simulink model "Coupled_Model_crosslinked_intext"  (R2016a)
settings: Solver=FixedStepDiscrete  StartTime=0  StopTime=1000  FixedStep=1  RelTol=1e-3
undefined symbols (not defined in the file or in its folder): DiscIntNeverNeededParam
libraries: simulink_extras x32
(part 2 of 3)

== system Coupled_Model_crosslinked_intext/kMtcontrol/kMtcontrol3/kMt Dynamics ==
  Fk : Inport
  Add : Sum  Inputs=-+
  Add1 : Sum  Inputs=-+
  Add2 : Sum
  Discrete-Time Integrator : DiscreteIntegrator  InitialConditionSource=external  ICPrevOutput=DiscIntNeverNeededParam  ICPrevScaledInput=DiscIntNeverNeededParam
  Discrete-Time Integrator1 : DiscreteIntegrator  InitialConditionSource=external  ICPrevOutput=DiscIntNeverNeededParam  ICPrevScaledInput=DiscIntNeverNeededParam
  Mux : Mux  Inputs=2
  Product{1..4} (4 alike) : Product  RndMeth=Zero
  kMtState : Subsystem
  LkMt : Outport
  tag scope: kMt13=global
  wires:
  Fk/1 -> kMtState/2(Fspr)
  kMtState/2(RLeft) -> Product2/1
  Product1/1 -> Add/1
  Product2/1 -> Add/2
  Product3/1 -> Add1/2
  Product4/1 -> Add1/1
  kMtState/4(RRight) -> Product3/1
  kMtState/1(CLeft) -> Product1/1
  Add/1 -> Discrete-Time Integrator/1  "glkMt"
  Add1/1 -> Discrete-Time Integrator1/1  "grkMt"
  Discrete-Time Integrator1/1 -> Add2/2, kMtState/3(LrkMt), Mux/2
  Discrete-Time Integrator/1 -> Add2/1, kMtState/1(LlkMt), Mux/1
  Add2/1 -> LkMt/1
  kMtState/3(CRight) -> Product4/1
  [Rgro] -> Product2/2, Product3/2
  [Rshr] -> Product1/2, Product4/2
  Mux/1 -> [kMt13]
  [LkMt] -> Discrete-Time Integrator/2
  [LkMt] -> Discrete-Time Integrator1/2

== system Coupled_Model_crosslinked_intext/kMtcontrol/kMtcontrol3/kMt Dynamics  ==
  Fk : Inport
  Add : Sum  Inputs=-+
  Add1 : Sum  Inputs=-+
  Add2 : Sum
  Discrete-Time Integrator : DiscreteIntegrator  InitialConditionSource=external  ICPrevOutput=DiscIntNeverNeededParam  ICPrevScaledInput=DiscIntNeverNeededParam
  Discrete-Time Integrator1 : DiscreteIntegrator  InitialConditionSource=external  ICPrevOutput=DiscIntNeverNeededParam  ICPrevScaledInput=DiscIntNeverNeededParam
  Mux : Mux  Inputs=2
  Product{1..4} (4 alike) : Product  RndMeth=Zero
  kMtState : Subsystem
  LkMt : Outport
  tag scope: kMt14=global
  wires:
  Fk/1 -> kMtState/2(Fspr)
  kMtState/2(RLeft) -> Product2/1
  Product1/1 -> Add/1
  Product2/1 -> Add/2
  Product3/1 -> Add1/2
  Product4/1 -> Add1/1
  kMtState/4(RRight) -> Product3/1
  kMtState/1(CLeft) -> Product1/1
  Add/1 -> Discrete-Time Integrator/1  "glkMt"
  Add1/1 -> Discrete-Time Integrator1/1  "grkMt"
  Discrete-Time Integrator1/1 -> Add2/2, kMtState/3(LrkMt), Mux/2
  Discrete-Time Integrator/1 -> Add2/1, kMtState/1(LlkMt), Mux/1
  Add2/1 -> LkMt/1
  kMtState/3(CRight) -> Product4/1
  [Rgro] -> Product2/2, Product3/2
  [Rshr] -> Product1/2, Product4/2
  Mux/1 -> [kMt14]
  [LkMt] -> Discrete-Time Integrator/2
  [LkMt] -> Discrete-Time Integrator1/2

== system Coupled_Model_crosslinked_intext/kMtcontrol/kMtcontrol3/kMt Dynamics   ==
  Fk : Inport
  Add : Sum  Inputs=-+
  Add1 : Sum  Inputs=-+
  Add2 : Sum
  Discrete-Time Integrator : DiscreteIntegrator  InitialConditionSource=external  ICPrevOutput=DiscIntNeverNeededParam  ICPrevScaledInput=DiscIntNeverNeededParam
  Discrete-Time Integrator1 : DiscreteIntegrator  InitialConditionSource=external  ICPrevOutput=DiscIntNeverNeededParam  ICPrevScaledInput=DiscIntNeverNeededParam
  Mux : Mux  Inputs=2
  Product{1..4} (4 alike) : Product  RndMeth=Zero
  kMtState : Subsystem
  LkMt : Outport
  tag scope: kMt16=global
  wires:
  Fk/1 -> kMtState/2(Fspr)
  kMtState/2(RLeft) -> Product2/1
  Product1/1 -> Add/1
  Product2/1 -> Add/2
  Product3/1 -> Add1/2
  Product4/1 -> Add1/1
  kMtState/4(RRight) -> Product3/1
  kMtState/1(CLeft) -> Product1/1
  Add/1 -> Discrete-Time Integrator/1  "glkMt"
  Add1/1 -> Discrete-Time Integrator1/1  "grkMt"
  Discrete-Time Integrator1/1 -> Add2/2, kMtState/3(LrkMt), Mux/2
  Discrete-Time Integrator/1 -> Add2/1, kMtState/1(LlkMt), Mux/1
  Add2/1 -> LkMt/1
  kMtState/3(CRight) -> Product4/1
  [Rgro] -> Product2/2, Product3/2
  [Rshr] -> Product1/2, Product4/2
  Mux/1 -> [kMt16]
  [LkMt] -> Discrete-Time Integrator/2
  [LkMt] -> Discrete-Time Integrator1/2

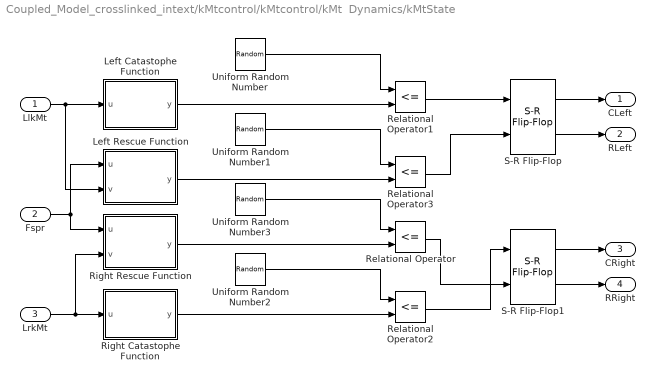
== system Coupled_Model_crosslinked_intext/kMtcontrol/kMtcontrol/kMt  Dynamics/kMtState ==
  LlkMt : Inport
  Fspr : Inport  Port=2
  LrkMt : Inport  Port=3
  Left Catastophe Function : MATLAB Function  TreatAsAtomicUnit=on
  Left Rescue Function : MATLAB Function  TreatAsAtomicUnit=on
  Relational Operator{,1..3} (4 alike) : RelationalOperator  Operator=<=  OutDataTypeStr=boolean
  Right Catastophe Function : MATLAB Function  TreatAsAtomicUnit=on
  Right Rescue Function : MATLAB Function  TreatAsAtomicUnit=on
  S-R Flip-Flop : simulink_extras/Flip Flops/S-R Flip-Flop  SystemSampleTime=-1  initial_condition=0
  S-R Flip-Flop1 : simulink_extras/Flip Flops/S-R Flip-Flop  SystemSampleTime=-1  initial_condition=0
  Uniform Random Number : UniformRandomNumber  Minimum=0  Seed=randi(10000)+1  SampleTime=1
  Uniform Random Number1 : UniformRandomNumber  Minimum=0  Seed=randi(10000)+2  SampleTime=1
  Uniform Random Number2 : UniformRandomNumber  Minimum=0  Seed=randi(10000)+4  SampleTime=1
  Uniform Random Number3 : UniformRandomNumber  Minimum=0  Seed=randi(10000)+3  SampleTime=1
  CLeft : Outport
  RLeft : Outport  Port=2
  CRight : Outport  Port=3
  RRight : Outport  Port=4
  wires:
  Left Catastophe Function/1(y) -> Relational Operator1/2
  Uniform Random Number/1 -> Relational Operator1/1
  Relational Operator1/1 -> S-R Flip-Flop/1
  Right Catastophe Function/1(y) -> Relational Operator2/2
  Uniform Random Number2/1 -> Relational Operator2/1
  Relational Operator2/1 -> S-R Flip-Flop1/1
  Uniform Random Number1/1 -> Relational Operator3/1
  Uniform Random Number3/1 -> Relational Operator/1
  Relational Operator3/1 -> S-R Flip-Flop/2
  Relational Operator/1 -> S-R Flip-Flop1/2
  Right Rescue Function/1(y) -> Relational Operator/2
  Left Rescue Function/1(y) -> Relational Operator3/2
  LlkMt/1 -> Left Catastophe Function/1(u), Left Rescue Function/2(v)
  LrkMt/1 -> Right Catastophe Function/1(u), Right Rescue Function/2(v)
  Fspr/1 -> Left Rescue Function/1(u), Right Rescue Function/1(u)
  S-R Flip-Flop/1 -> CLeft/1
  S-R Flip-Flop/2 -> RLeft/1
  S-R Flip-Flop1/1 -> CRight/1
  S-R Flip-Flop1/2 -> RRight/1

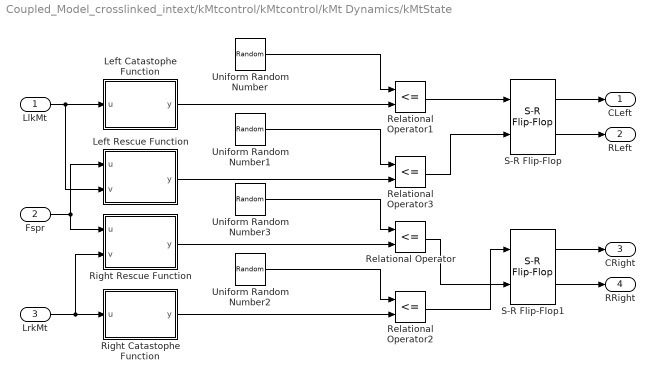
== system Coupled_Model_crosslinked_intext/kMtcontrol/kMtcontrol/kMt Dynamics/kMtState ==
  LlkMt : Inport
  Fspr : Inport  Port=2
  LrkMt : Inport  Port=3
  Left Catastophe Function : MATLAB Function  TreatAsAtomicUnit=on
  Left Rescue Function : MATLAB Function  TreatAsAtomicUnit=on
  Relational Operator{,1..3} (4 alike) : RelationalOperator  Operator=<=  OutDataTypeStr=boolean
  Right Catastophe Function : MATLAB Function  TreatAsAtomicUnit=on
  Right Rescue Function : MATLAB Function  TreatAsAtomicUnit=on
  S-R Flip-Flop : simulink_extras/Flip Flops/S-R Flip-Flop  SystemSampleTime=-1  initial_condition=0
  S-R Flip-Flop1 : simulink_extras/Flip Flops/S-R Flip-Flop  SystemSampleTime=-1  initial_condition=0
  Uniform Random Number : UniformRandomNumber  Minimum=0  Seed=randi(10000)+1  SampleTime=1
  Uniform Random Number1 : UniformRandomNumber  Minimum=0  Seed=randi(10000)+2  SampleTime=1
  Uniform Random Number2 : UniformRandomNumber  Minimum=0  Seed=randi(10000)+4  SampleTime=1
  Uniform Random Number3 : UniformRandomNumber  Minimum=0  Seed=randi(10000)+3  SampleTime=1
  CLeft : Outport
  RLeft : Outport  Port=2
  CRight : Outport  Port=3
  RRight : Outport  Port=4
  wires:
  Left Catastophe Function/1(y) -> Relational Operator1/2
  Uniform Random Number/1 -> Relational Operator1/1
  Relational Operator1/1 -> S-R Flip-Flop/1
  Right Catastophe Function/1(y) -> Relational Operator2/2
  Uniform Random Number2/1 -> Relational Operator2/1
  Relational Operator2/1 -> S-R Flip-Flop1/1
  Uniform Random Number1/1 -> Relational Operator3/1
  Uniform Random Number3/1 -> Relational Operator/1
  Relational Operator3/1 -> S-R Flip-Flop/2
  Relational Operator/1 -> S-R Flip-Flop1/2
  Right Rescue Function/1(y) -> Relational Operator/2
  Left Rescue Function/1(y) -> Relational Operator3/2
  LlkMt/1 -> Left Catastophe Function/1(u), Left Rescue Function/2(v)
  LrkMt/1 -> Right Catastophe Function/1(u), Right Rescue Function/2(v)
  Fspr/1 -> Left Rescue Function/1(u), Right Rescue Function/1(u)
  S-R Flip-Flop/1 -> CLeft/1
  S-R Flip-Flop/2 -> RLeft/1
  S-R Flip-Flop1/1 -> CRight/1
  S-R Flip-Flop1/2 -> RRight/1

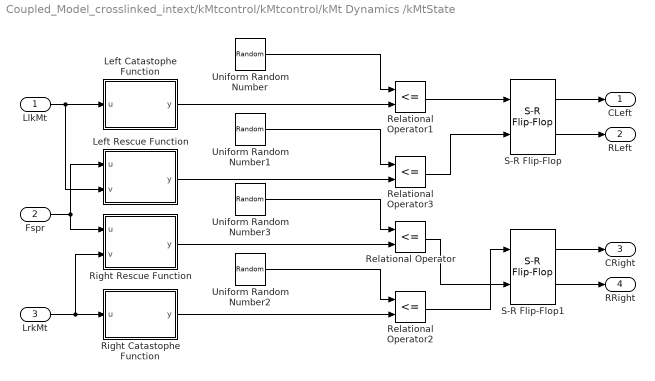
== system Coupled_Model_crosslinked_intext/kMtcontrol/kMtcontrol/kMt Dynamics /kMtState ==
  LlkMt : Inport
  Fspr : Inport  Port=2
  LrkMt : Inport  Port=3
  Left Catastophe Function : MATLAB Function  TreatAsAtomicUnit=on
  Left Rescue Function : MATLAB Function  TreatAsAtomicUnit=on
  Relational Operator{,1..3} (4 alike) : RelationalOperator  Operator=<=  OutDataTypeStr=boolean
  Right Catastophe Function : MATLAB Function  TreatAsAtomicUnit=on
  Right Rescue Function : MATLAB Function  TreatAsAtomicUnit=on
  S-R Flip-Flop : simulink_extras/Flip Flops/S-R Flip-Flop  SystemSampleTime=-1  initial_condition=0
  S-R Flip-Flop1 : simulink_extras/Flip Flops/S-R Flip-Flop  SystemSampleTime=-1  initial_condition=0
  Uniform Random Number : UniformRandomNumber  Minimum=0  Seed=randi(10000)+1  SampleTime=1
  Uniform Random Number1 : UniformRandomNumber  Minimum=0  Seed=randi(10000)+2  SampleTime=1
  Uniform Random Number2 : UniformRandomNumber  Minimum=0  Seed=randi(10000)+4  SampleTime=1
  Uniform Random Number3 : UniformRandomNumber  Minimum=0  Seed=randi(10000)+3  SampleTime=1
  CLeft : Outport
  RLeft : Outport  Port=2
  CRight : Outport  Port=3
  RRight : Outport  Port=4
  wires:
  Left Catastophe Function/1(y) -> Relational Operator1/2
  Uniform Random Number/1 -> Relational Operator1/1
  Relational Operator1/1 -> S-R Flip-Flop/1
  Right Catastophe Function/1(y) -> Relational Operator2/2
  Uniform Random Number2/1 -> Relational Operator2/1
  Relational Operator2/1 -> S-R Flip-Flop1/1
  Uniform Random Number1/1 -> Relational Operator3/1
  Uniform Random Number3/1 -> Relational Operator/1
  Relational Operator3/1 -> S-R Flip-Flop/2
  Relational Operator/1 -> S-R Flip-Flop1/2
  Right Rescue Function/1(y) -> Relational Operator/2
  Left Rescue Function/1(y) -> Relational Operator3/2
  LlkMt/1 -> Left Catastophe Function/1(u), Left Rescue Function/2(v)
  LrkMt/1 -> Right Catastophe Function/1(u), Right Rescue Function/2(v)
  Fspr/1 -> Left Rescue Function/1(u), Right Rescue Function/1(u)
  S-R Flip-Flop/1 -> CLeft/1
  S-R Flip-Flop/2 -> RLeft/1
  S-R Flip-Flop1/1 -> CRight/1
  S-R Flip-Flop1/2 -> RRight/1

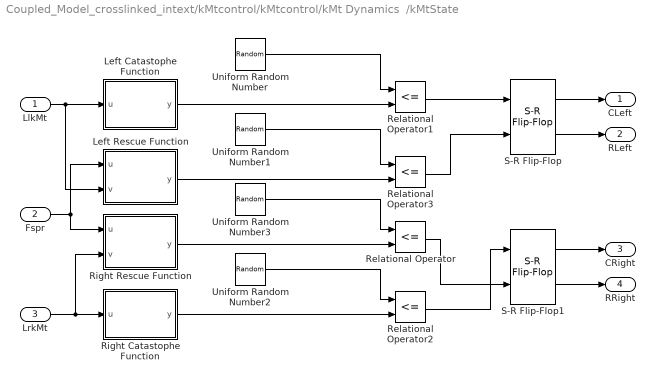
== system Coupled_Model_crosslinked_intext/kMtcontrol/kMtcontrol/kMt Dynamics  /kMtState ==
  LlkMt : Inport
  Fspr : Inport  Port=2
  LrkMt : Inport  Port=3
  Left Catastophe Function : MATLAB Function  TreatAsAtomicUnit=on
  Left Rescue Function : MATLAB Function  TreatAsAtomicUnit=on
  Relational Operator{,1..3} (4 alike) : RelationalOperator  Operator=<=  OutDataTypeStr=boolean
  Right Catastophe Function : MATLAB Function  TreatAsAtomicUnit=on
  Right Rescue Function : MATLAB Function  TreatAsAtomicUnit=on
  S-R Flip-Flop : simulink_extras/Flip Flops/S-R Flip-Flop  SystemSampleTime=-1  initial_condition=0
  S-R Flip-Flop1 : simulink_extras/Flip Flops/S-R Flip-Flop  SystemSampleTime=-1  initial_condition=0
  Uniform Random Number : UniformRandomNumber  Minimum=0  Seed=randi(10000)+1  SampleTime=1
  Uniform Random Number1 : UniformRandomNumber  Minimum=0  Seed=randi(10000)+2  SampleTime=1
  Uniform Random Number2 : UniformRandomNumber  Minimum=0  Seed=randi(10000)+4  SampleTime=1
  Uniform Random Number3 : UniformRandomNumber  Minimum=0  Seed=randi(10000)+3  SampleTime=1
  CLeft : Outport
  RLeft : Outport  Port=2
  CRight : Outport  Port=3
  RRight : Outport  Port=4
  wires:
  Left Catastophe Function/1(y) -> Relational Operator1/2
  Uniform Random Number/1 -> Relational Operator1/1
  Relational Operator1/1 -> S-R Flip-Flop/1
  Right Catastophe Function/1(y) -> Relational Operator2/2
  Uniform Random Number2/1 -> Relational Operator2/1
  Relational Operator2/1 -> S-R Flip-Flop1/1
  Uniform Random Number1/1 -> Relational Operator3/1
  Uniform Random Number3/1 -> Relational Operator/1
  Relational Operator3/1 -> S-R Flip-Flop/2
  Relational Operator/1 -> S-R Flip-Flop1/2
  Right Rescue Function/1(y) -> Relational Operator/2
  Left Rescue Function/1(y) -> Relational Operator3/2
  LlkMt/1 -> Left Catastophe Function/1(u), Left Rescue Function/2(v)
  LrkMt/1 -> Right Catastophe Function/1(u), Right Rescue Function/2(v)
  Fspr/1 -> Left Rescue Function/1(u), Right Rescue Function/1(u)
  S-R Flip-Flop/1 -> CLeft/1
  S-R Flip-Flop/2 -> RLeft/1
  S-R Flip-Flop1/1 -> CRight/1
  S-R Flip-Flop1/2 -> RRight/1

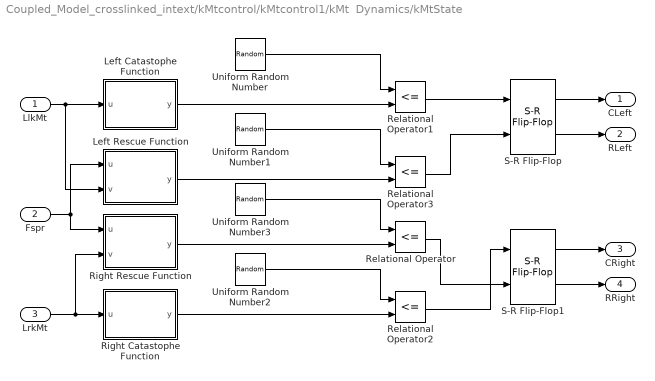
== system Coupled_Model_crosslinked_intext/kMtcontrol/kMtcontrol1/kMt  Dynamics/kMtState ==
  LlkMt : Inport
  Fspr : Inport  Port=2
  LrkMt : Inport  Port=3
  Left Catastophe Function : MATLAB Function  TreatAsAtomicUnit=on
  Left Rescue Function : MATLAB Function  TreatAsAtomicUnit=on
  Relational Operator{,1..3} (4 alike) : RelationalOperator  Operator=<=  OutDataTypeStr=boolean
  Right Catastophe Function : MATLAB Function  TreatAsAtomicUnit=on
  Right Rescue Function : MATLAB Function  TreatAsAtomicUnit=on
  S-R Flip-Flop : simulink_extras/Flip Flops/S-R Flip-Flop  SystemSampleTime=-1  initial_condition=0
  S-R Flip-Flop1 : simulink_extras/Flip Flops/S-R Flip-Flop  SystemSampleTime=-1  initial_condition=0
  Uniform Random Number : UniformRandomNumber  Minimum=0  Seed=randi(10000)+1  SampleTime=1
  Uniform Random Number1 : UniformRandomNumber  Minimum=0  Seed=randi(10000)+2  SampleTime=1
  Uniform Random Number2 : UniformRandomNumber  Minimum=0  Seed=randi(10000)+4  SampleTime=1
  Uniform Random Number3 : UniformRandomNumber  Minimum=0  Seed=randi(10000)+3  SampleTime=1
  CLeft : Outport
  RLeft : Outport  Port=2
  CRight : Outport  Port=3
  RRight : Outport  Port=4
  wires:
  Left Catastophe Function/1(y) -> Relational Operator1/2
  Uniform Random Number/1 -> Relational Operator1/1
  Relational Operator1/1 -> S-R Flip-Flop/1
  Right Catastophe Function/1(y) -> Relational Operator2/2
  Uniform Random Number2/1 -> Relational Operator2/1
  Relational Operator2/1 -> S-R Flip-Flop1/1
  Uniform Random Number1/1 -> Relational Operator3/1
  Uniform Random Number3/1 -> Relational Operator/1
  Relational Operator3/1 -> S-R Flip-Flop/2
  Relational Operator/1 -> S-R Flip-Flop1/2
  Right Rescue Function/1(y) -> Relational Operator/2
  Left Rescue Function/1(y) -> Relational Operator3/2
  LlkMt/1 -> Left Catastophe Function/1(u), Left Rescue Function/2(v)
  LrkMt/1 -> Right Catastophe Function/1(u), Right Rescue Function/2(v)
  Fspr/1 -> Left Rescue Function/1(u), Right Rescue Function/1(u)
  S-R Flip-Flop/1 -> CLeft/1
  S-R Flip-Flop/2 -> RLeft/1
  S-R Flip-Flop1/1 -> CRight/1
  S-R Flip-Flop1/2 -> RRight/1

== system Coupled_Model_crosslinked_intext/kMtcontrol/kMtcontrol1/kMt Dynamics/kMtState ==
  LlkMt : Inport
  Fspr : Inport  Port=2
  LrkMt : Inport  Port=3
  Left Catastophe Function : MATLAB Function  TreatAsAtomicUnit=on
  Left Rescue Function : MATLAB Function  TreatAsAtomicUnit=on
  Relational Operator{,1..3} (4 alike) : RelationalOperator  Operator=<=  OutDataTypeStr=boolean
  Right Catastophe Function : MATLAB Function  TreatAsAtomicUnit=on
  Right Rescue Function : MATLAB Function  TreatAsAtomicUnit=on
  S-R Flip-Flop : simulink_extras/Flip Flops/S-R Flip-Flop  SystemSampleTime=-1  initial_condition=0
  S-R Flip-Flop1 : simulink_extras/Flip Flops/S-R Flip-Flop  SystemSampleTime=-1  initial_condition=0
  Uniform Random Number : UniformRandomNumber  Minimum=0  Seed=randi(10000)+1  SampleTime=1
  Uniform Random Number1 : UniformRandomNumber  Minimum=0  Seed=randi(10000)+2  SampleTime=1
  Uniform Random Number2 : UniformRandomNumber  Minimum=0  Seed=randi(10000)+4  SampleTime=1
  Uniform Random Number3 : UniformRandomNumber  Minimum=0  Seed=randi(10000)+3  SampleTime=1
  CLeft : Outport
  RLeft : Outport  Port=2
  CRight : Outport  Port=3
  RRight : Outport  Port=4
  wires:
  Left Catastophe Function/1(y) -> Relational Operator1/2
  Uniform Random Number/1 -> Relational Operator1/1
  Relational Operator1/1 -> S-R Flip-Flop/1
  Right Catastophe Function/1(y) -> Relational Operator2/2
  Uniform Random Number2/1 -> Relational Operator2/1
  Relational Operator2/1 -> S-R Flip-Flop1/1
  Uniform Random Number1/1 -> Relational Operator3/1
  Uniform Random Number3/1 -> Relational Operator/1
  Relational Operator3/1 -> S-R Flip-Flop/2
  Relational Operator/1 -> S-R Flip-Flop1/2
  Right Rescue Function/1(y) -> Relational Operator/2
  Left Rescue Function/1(y) -> Relational Operator3/2
  LlkMt/1 -> Left Catastophe Function/1(u), Left Rescue Function/2(v)
  LrkMt/1 -> Right Catastophe Function/1(u), Right Rescue Function/2(v)
  Fspr/1 -> Left Rescue Function/1(u), Right Rescue Function/1(u)
  S-R Flip-Flop/1 -> CLeft/1
  S-R Flip-Flop/2 -> RLeft/1
  S-R Flip-Flop1/1 -> CRight/1
  S-R Flip-Flop1/2 -> RRight/1

== system Coupled_Model_crosslinked_intext/kMtcontrol/kMtcontrol1/kMt Dynamics /kMtState ==
  LlkMt : Inport
  Fspr : Inport  Port=2
  LrkMt : Inport  Port=3
  Left Catastophe Function : MATLAB Function  TreatAsAtomicUnit=on
  Left Rescue Function : MATLAB Function  TreatAsAtomicUnit=on
  Relational Operator{,1..3} (4 alike) : RelationalOperator  Operator=<=  OutDataTypeStr=boolean
  Right Catastophe Function : MATLAB Function  TreatAsAtomicUnit=on
  Right Rescue Function : MATLAB Function  TreatAsAtomicUnit=on
  S-R Flip-Flop : simulink_extras/Flip Flops/S-R Flip-Flop  SystemSampleTime=-1  initial_condition=0
  S-R Flip-Flop1 : simulink_extras/Flip Flops/S-R Flip-Flop  SystemSampleTime=-1  initial_condition=0
  Uniform Random Number : UniformRandomNumber  Minimum=0  Seed=randi(10000)+1  SampleTime=1
  Uniform Random Number1 : UniformRandomNumber  Minimum=0  Seed=randi(10000)+2  SampleTime=1
  Uniform Random Number2 : UniformRandomNumber  Minimum=0  Seed=randi(10000)+4  SampleTime=1
  Uniform Random Number3 : UniformRandomNumber  Minimum=0  Seed=randi(10000)+3  SampleTime=1
  CLeft : Outport
  RLeft : Outport  Port=2
  CRight : Outport  Port=3
  RRight : Outport  Port=4
  wires:
  Left Catastophe Function/1(y) -> Relational Operator1/2
  Uniform Random Number/1 -> Relational Operator1/1
  Relational Operator1/1 -> S-R Flip-Flop/1
  Right Catastophe Function/1(y) -> Relational Operator2/2
  Uniform Random Number2/1 -> Relational Operator2/1
  Relational Operator2/1 -> S-R Flip-Flop1/1
  Uniform Random Number1/1 -> Relational Operator3/1
  Uniform Random Number3/1 -> Relational Operator/1
  Relational Operator3/1 -> S-R Flip-Flop/2
  Relational Operator/1 -> S-R Flip-Flop1/2
  Right Rescue Function/1(y) -> Relational Operator/2
  Left Rescue Function/1(y) -> Relational Operator3/2
  LlkMt/1 -> Left Catastophe Function/1(u), Left Rescue Function/2(v)
  LrkMt/1 -> Right Catastophe Function/1(u), Right Rescue Function/2(v)
  Fspr/1 -> Left Rescue Function/1(u), Right Rescue Function/1(u)
  S-R Flip-Flop/1 -> CLeft/1
  S-R Flip-Flop/2 -> RLeft/1
  S-R Flip-Flop1/1 -> CRight/1
  S-R Flip-Flop1/2 -> RRight/1

== system Coupled_Model_crosslinked_intext/kMtcontrol/kMtcontrol1/kMt Dynamics  /kMtState ==
  LlkMt : Inport
  Fspr : Inport  Port=2
  LrkMt : Inport  Port=3
  Left Catastophe Function : MATLAB Function  TreatAsAtomicUnit=on
  Left Rescue Function : MATLAB Function  TreatAsAtomicUnit=on
  Relational Operator{,1..3} (4 alike) : RelationalOperator  Operator=<=  OutDataTypeStr=boolean
  Right Catastophe Function : MATLAB Function  TreatAsAtomicUnit=on
  Right Rescue Function : MATLAB Function  TreatAsAtomicUnit=on
  S-R Flip-Flop : simulink_extras/Flip Flops/S-R Flip-Flop  SystemSampleTime=-1  initial_condition=0
  S-R Flip-Flop1 : simulink_extras/Flip Flops/S-R Flip-Flop  SystemSampleTime=-1  initial_condition=0
  Uniform Random Number : UniformRandomNumber  Minimum=0  Seed=randi(10000)+1  SampleTime=1
  Uniform Random Number1 : UniformRandomNumber  Minimum=0  Seed=randi(10000)+2  SampleTime=1
  Uniform Random Number2 : UniformRandomNumber  Minimum=0  Seed=randi(10000)+4  SampleTime=1
  Uniform Random Number3 : UniformRandomNumber  Minimum=0  Seed=randi(10000)+3  SampleTime=1
  CLeft : Outport
  RLeft : Outport  Port=2
  CRight : Outport  Port=3
  RRight : Outport  Port=4
  wires:
  Left Catastophe Function/1(y) -> Relational Operator1/2
  Uniform Random Number/1 -> Relational Operator1/1
  Relational Operator1/1 -> S-R Flip-Flop/1
  Right Catastophe Function/1(y) -> Relational Operator2/2
  Uniform Random Number2/1 -> Relational Operator2/1
  Relational Operator2/1 -> S-R Flip-Flop1/1
  Uniform Random Number1/1 -> Relational Operator3/1
  Uniform Random Number3/1 -> Relational Operator/1
  Relational Operator3/1 -> S-R Flip-Flop/2
  Relational Operator/1 -> S-R Flip-Flop1/2
  Right Rescue Function/1(y) -> Relational Operator/2
  Left Rescue Function/1(y) -> Relational Operator3/2
  LlkMt/1 -> Left Catastophe Function/1(u), Left Rescue Function/2(v)
  LrkMt/1 -> Right Catastophe Function/1(u), Right Rescue Function/2(v)
  Fspr/1 -> Left Rescue Function/1(u), Right Rescue Function/1(u)
  S-R Flip-Flop/1 -> CLeft/1
  S-R Flip-Flop/2 -> RLeft/1
  S-R Flip-Flop1/1 -> CRight/1
  S-R Flip-Flop1/2 -> RRight/1

== system Coupled_Model_crosslinked_intext/kMtcontrol/kMtcontrol2/kMt  Dynamics/kMtState ==
  LlkMt : Inport
  Fspr : Inport  Port=2
  LrkMt : Inport  Port=3
  Left Catastophe Function : MATLAB Function  TreatAsAtomicUnit=on
  Left Rescue Function : MATLAB Function  TreatAsAtomicUnit=on
  Relational Operator{,1..3} (4 alike) : RelationalOperator  Operator=<=  OutDataTypeStr=boolean
  Right Catastophe Function : MATLAB Function  TreatAsAtomicUnit=on
  Right Rescue Function : MATLAB Function  TreatAsAtomicUnit=on
  S-R Flip-Flop : simulink_extras/Flip Flops/S-R Flip-Flop  SystemSampleTime=-1  initial_condition=0
  S-R Flip-Flop1 : simulink_extras/Flip Flops/S-R Flip-Flop  SystemSampleTime=-1  initial_condition=0
  Uniform Random Number : UniformRandomNumber  Minimum=0  Seed=randi(10000)+1  SampleTime=1
  Uniform Random Number1 : UniformRandomNumber  Minimum=0  Seed=randi(10000)+2  SampleTime=1
  Uniform Random Number2 : UniformRandomNumber  Minimum=0  Seed=randi(10000)+4  SampleTime=1
  Uniform Random Number3 : UniformRandomNumber  Minimum=0  Seed=randi(10000)+3  SampleTime=1
  CLeft : Outport
  RLeft : Outport  Port=2
  CRight : Outport  Port=3
  RRight : Outport  Port=4
  wires:
  Left Catastophe Function/1(y) -> Relational Operator1/2
  Uniform Random Number/1 -> Relational Operator1/1
  Relational Operator1/1 -> S-R Flip-Flop/1
  Right Catastophe Function/1(y) -> Relational Operator2/2
  Uniform Random Number2/1 -> Relational Operator2/1
  Relational Operator2/1 -> S-R Flip-Flop1/1
  Uniform Random Number1/1 -> Relational Operator3/1
  Uniform Random Number3/1 -> Relational Operator/1
  Relational Operator3/1 -> S-R Flip-Flop/2
  Relational Operator/1 -> S-R Flip-Flop1/2
  Right Rescue Function/1(y) -> Relational Operator/2
  Left Rescue Function/1(y) -> Relational Operator3/2
  LlkMt/1 -> Left Catastophe Function/1(u), Left Rescue Function/2(v)
  LrkMt/1 -> Right Catastophe Function/1(u), Right Rescue Function/2(v)
  Fspr/1 -> Left Rescue Function/1(u), Right Rescue Function/1(u)
  S-R Flip-Flop/1 -> CLeft/1
  S-R Flip-Flop/2 -> RLeft/1
  S-R Flip-Flop1/1 -> CRight/1
  S-R Flip-Flop1/2 -> RRight/1

== system Coupled_Model_crosslinked_intext/kMtcontrol/kMtcontrol2/kMt Dynamics/kMtState ==
  LlkMt : Inport
  Fspr : Inport  Port=2
  LrkMt : Inport  Port=3
  Left Catastophe Function : MATLAB Function  TreatAsAtomicUnit=on
  Left Rescue Function : MATLAB Function  TreatAsAtomicUnit=on
  Relational Operator{,1..3} (4 alike) : RelationalOperator  Operator=<=  OutDataTypeStr=boolean
  Right Catastophe Function : MATLAB Function  TreatAsAtomicUnit=on
  Right Rescue Function : MATLAB Function  TreatAsAtomicUnit=on
  S-R Flip-Flop : simulink_extras/Flip Flops/S-R Flip-Flop  SystemSampleTime=-1  initial_condition=0
  S-R Flip-Flop1 : simulink_extras/Flip Flops/S-R Flip-Flop  SystemSampleTime=-1  initial_condition=0
  Uniform Random Number : UniformRandomNumber  Minimum=0  Seed=randi(10000)+1  SampleTime=1
  Uniform Random Number1 : UniformRandomNumber  Minimum=0  Seed=randi(10000)+2  SampleTime=1
  Uniform Random Number2 : UniformRandomNumber  Minimum=0  Seed=randi(10000)+4  SampleTime=1
  Uniform Random Number3 : UniformRandomNumber  Minimum=0  Seed=randi(10000)+3  SampleTime=1
  CLeft : Outport
  RLeft : Outport  Port=2
  CRight : Outport  Port=3
  RRight : Outport  Port=4
  wires:
  Left Catastophe Function/1(y) -> Relational Operator1/2
  Uniform Random Number/1 -> Relational Operator1/1
  Relational Operator1/1 -> S-R Flip-Flop/1
  Right Catastophe Function/1(y) -> Relational Operator2/2
  Uniform Random Number2/1 -> Relational Operator2/1
  Relational Operator2/1 -> S-R Flip-Flop1/1
  Uniform Random Number1/1 -> Relational Operator3/1
  Uniform Random Number3/1 -> Relational Operator/1
  Relational Operator3/1 -> S-R Flip-Flop/2
  Relational Operator/1 -> S-R Flip-Flop1/2
  Right Rescue Function/1(y) -> Relational Operator/2
  Left Rescue Function/1(y) -> Relational Operator3/2
  LlkMt/1 -> Left Catastophe Function/1(u), Left Rescue Function/2(v)
  LrkMt/1 -> Right Catastophe Function/1(u), Right Rescue Function/2(v)
  Fspr/1 -> Left Rescue Function/1(u), Right Rescue Function/1(u)
  S-R Flip-Flop/1 -> CLeft/1
  S-R Flip-Flop/2 -> RLeft/1
  S-R Flip-Flop1/1 -> CRight/1
  S-R Flip-Flop1/2 -> RRight/1

== system Coupled_Model_crosslinked_intext/kMtcontrol/kMtcontrol2/kMt Dynamics /kMtState ==
  LlkMt : Inport
  Fspr : Inport  Port=2
  LrkMt : Inport  Port=3
  Left Catastophe Function : MATLAB Function  TreatAsAtomicUnit=on
  Left Rescue Function : MATLAB Function  TreatAsAtomicUnit=on
  Relational Operator{,1..3} (4 alike) : RelationalOperator  Operator=<=  OutDataTypeStr=boolean
  Right Catastophe Function : MATLAB Function  TreatAsAtomicUnit=on
  Right Rescue Function : MATLAB Function  TreatAsAtomicUnit=on
  S-R Flip-Flop : simulink_extras/Flip Flops/S-R Flip-Flop  SystemSampleTime=-1  initial_condition=0
  S-R Flip-Flop1 : simulink_extras/Flip Flops/S-R Flip-Flop  SystemSampleTime=-1  initial_condition=0
  Uniform Random Number : UniformRandomNumber  Minimum=0  Seed=randi(10000)+1  SampleTime=1
  Uniform Random Number1 : UniformRandomNumber  Minimum=0  Seed=randi(10000)+2  SampleTime=1
  Uniform Random Number2 : UniformRandomNumber  Minimum=0  Seed=randi(10000)+4  SampleTime=1
  Uniform Random Number3 : UniformRandomNumber  Minimum=0  Seed=randi(10000)+3  SampleTime=1
  CLeft : Outport
  RLeft : Outport  Port=2
  CRight : Outport  Port=3
  RRight : Outport  Port=4
  wires:
  Left Catastophe Function/1(y) -> Relational Operator1/2
  Uniform Random Number/1 -> Relational Operator1/1
  Relational Operator1/1 -> S-R Flip-Flop/1
  Right Catastophe Function/1(y) -> Relational Operator2/2
  Uniform Random Number2/1 -> Relational Operator2/1
  Relational Operator2/1 -> S-R Flip-Flop1/1
  Uniform Random Number1/1 -> Relational Operator3/1
  Uniform Random Number3/1 -> Relational Operator/1
  Relational Operator3/1 -> S-R Flip-Flop/2
  Relational Operator/1 -> S-R Flip-Flop1/2
  Right Rescue Function/1(y) -> Relational Operator/2
  Left Rescue Function/1(y) -> Relational Operator3/2
  LlkMt/1 -> Left Catastophe Function/1(u), Left Rescue Function/2(v)
  LrkMt/1 -> Right Catastophe Function/1(u), Right Rescue Function/2(v)
  Fspr/1 -> Left Rescue Function/1(u), Right Rescue Function/1(u)
  S-R Flip-Flop/1 -> CLeft/1
  S-R Flip-Flop/2 -> RLeft/1
  S-R Flip-Flop1/1 -> CRight/1
  S-R Flip-Flop1/2 -> RRight/1

== system Coupled_Model_crosslinked_intext/kMtcontrol/kMtcontrol2/kMt Dynamics  /kMtState ==
  LlkMt : Inport
  Fspr : Inport  Port=2
  LrkMt : Inport  Port=3
  Left Catastophe Function : MATLAB Function  TreatAsAtomicUnit=on
  Left Rescue Function : MATLAB Function  TreatAsAtomicUnit=on
  Relational Operator{,1..3} (4 alike) : RelationalOperator  Operator=<=  OutDataTypeStr=boolean
  Right Catastophe Function : MATLAB Function  TreatAsAtomicUnit=on
  Right Rescue Function : MATLAB Function  TreatAsAtomicUnit=on
  S-R Flip-Flop : simulink_extras/Flip Flops/S-R Flip-Flop  SystemSampleTime=-1  initial_condition=0
  S-R Flip-Flop1 : simulink_extras/Flip Flops/S-R Flip-Flop  SystemSampleTime=-1  initial_condition=0
  Uniform Random Number : UniformRandomNumber  Minimum=0  Seed=randi(10000)+1  SampleTime=1
  Uniform Random Number1 : UniformRandomNumber  Minimum=0  Seed=randi(10000)+2  SampleTime=1
  Uniform Random Number2 : UniformRandomNumber  Minimum=0  Seed=randi(10000)+4  SampleTime=1
  Uniform Random Number3 : UniformRandomNumber  Minimum=0  Seed=randi(10000)+3  SampleTime=1
  CLeft : Outport
  RLeft : Outport  Port=2
  CRight : Outport  Port=3
  RRight : Outport  Port=4
  wires:
  Left Catastophe Function/1(y) -> Relational Operator1/2
  Uniform Random Number/1 -> Relational Operator1/1
  Relational Operator1/1 -> S-R Flip-Flop/1
  Right Catastophe Function/1(y) -> Relational Operator2/2
  Uniform Random Number2/1 -> Relational Operator2/1
  Relational Operator2/1 -> S-R Flip-Flop1/1
  Uniform Random Number1/1 -> Relational Operator3/1
  Uniform Random Number3/1 -> Relational Operator/1
  Relational Operator3/1 -> S-R Flip-Flop/2
  Relational Operator/1 -> S-R Flip-Flop1/2
  Right Rescue Function/1(y) -> Relational Operator/2
  Left Rescue Function/1(y) -> Relational Operator3/2
  LlkMt/1 -> Left Catastophe Function/1(u), Left Rescue Function/2(v)
  LrkMt/1 -> Right Catastophe Function/1(u), Right Rescue Function/2(v)
  Fspr/1 -> Left Rescue Function/1(u), Right Rescue Function/1(u)
  S-R Flip-Flop/1 -> CLeft/1
  S-R Flip-Flop/2 -> RLeft/1
  S-R Flip-Flop1/1 -> CRight/1
  S-R Flip-Flop1/2 -> RRight/1

== system Coupled_Model_crosslinked_intext/kMtcontrol/kMtcontrol3/kMt  Dynamics/kMtState ==
  LlkMt : Inport
  Fspr : Inport  Port=2
  LrkMt : Inport  Port=3
  Left Catastophe Function : MATLAB Function  TreatAsAtomicUnit=on
  Left Rescue Function : MATLAB Function  TreatAsAtomicUnit=on
  Relational Operator{,1..3} (4 alike) : RelationalOperator  Operator=<=  OutDataTypeStr=boolean
  Right Catastophe Function : MATLAB Function  TreatAsAtomicUnit=on
  Right Rescue Function : MATLAB Function  TreatAsAtomicUnit=on
  S-R Flip-Flop : simulink_extras/Flip Flops/S-R Flip-Flop  SystemSampleTime=-1  initial_condition=0
  S-R Flip-Flop1 : simulink_extras/Flip Flops/S-R Flip-Flop  SystemSampleTime=-1  initial_condition=0
  Uniform Random Number : UniformRandomNumber  Minimum=0  Seed=randi(10000)+1  SampleTime=1
  Uniform Random Number1 : UniformRandomNumber  Minimum=0  Seed=randi(10000)+2  SampleTime=1
  Uniform Random Number2 : UniformRandomNumber  Minimum=0  Seed=randi(10000)+4  SampleTime=1
  Uniform Random Number3 : UniformRandomNumber  Minimum=0  Seed=randi(10000)+3  SampleTime=1
  CLeft : Outport
  RLeft : Outport  Port=2
  CRight : Outport  Port=3
  RRight : Outport  Port=4
  wires:
  Left Catastophe Function/1(y) -> Relational Operator1/2
  Uniform Random Number/1 -> Relational Operator1/1
  Relational Operator1/1 -> S-R Flip-Flop/1
  Right Catastophe Function/1(y) -> Relational Operator2/2
  Uniform Random Number2/1 -> Relational Operator2/1
  Relational Operator2/1 -> S-R Flip-Flop1/1
  Uniform Random Number1/1 -> Relational Operator3/1
  Uniform Random Number3/1 -> Relational Operator/1
  Relational Operator3/1 -> S-R Flip-Flop/2
  Relational Operator/1 -> S-R Flip-Flop1/2
  Right Rescue Function/1(y) -> Relational Operator/2
  Left Rescue Function/1(y) -> Relational Operator3/2
  LlkMt/1 -> Left Catastophe Function/1(u), Left Rescue Function/2(v)
  LrkMt/1 -> Right Catastophe Function/1(u), Right Rescue Function/2(v)
  Fspr/1 -> Left Rescue Function/1(u), Right Rescue Function/1(u)
  S-R Flip-Flop/1 -> CLeft/1
  S-R Flip-Flop/2 -> RLeft/1
  S-R Flip-Flop1/1 -> CRight/1
  S-R Flip-Flop1/2 -> RRight/1

== system Coupled_Model_crosslinked_intext/kMtcontrol/kMtcontrol3/kMt Dynamics/kMtState ==
  LlkMt : Inport
  Fspr : Inport  Port=2
  LrkMt : Inport  Port=3
  Left Catastophe Function : MATLAB Function  TreatAsAtomicUnit=on
  Left Rescue Function : MATLAB Function  TreatAsAtomicUnit=on
  Relational Operator{,1..3} (4 alike) : RelationalOperator  Operator=<=  OutDataTypeStr=boolean
  Right Catastophe Function : MATLAB Function  TreatAsAtomicUnit=on
  Right Rescue Function : MATLAB Function  TreatAsAtomicUnit=on
  S-R Flip-Flop : simulink_extras/Flip Flops/S-R Flip-Flop  SystemSampleTime=-1  initial_condition=0
  S-R Flip-Flop1 : simulink_extras/Flip Flops/S-R Flip-Flop  SystemSampleTime=-1  initial_condition=0
  Uniform Random Number : UniformRandomNumber  Minimum=0  Seed=randi(10000)+1  SampleTime=1
  Uniform Random Number1 : UniformRandomNumber  Minimum=0  Seed=randi(10000)+2  SampleTime=1
  Uniform Random Number2 : UniformRandomNumber  Minimum=0  Seed=randi(10000)+4  SampleTime=1
  Uniform Random Number3 : UniformRandomNumber  Minimum=0  Seed=randi(10000)+3  SampleTime=1
  CLeft : Outport
  RLeft : Outport  Port=2
  CRight : Outport  Port=3
  RRight : Outport  Port=4
  wires:
  Left Catastophe Function/1(y) -> Relational Operator1/2
  Uniform Random Number/1 -> Relational Operator1/1
  Relational Operator1/1 -> S-R Flip-Flop/1
  Right Catastophe Function/1(y) -> Relational Operator2/2
  Uniform Random Number2/1 -> Relational Operator2/1
  Relational Operator2/1 -> S-R Flip-Flop1/1
  Uniform Random Number1/1 -> Relational Operator3/1
  Uniform Random Number3/1 -> Relational Operator/1
  Relational Operator3/1 -> S-R Flip-Flop/2
  Relational Operator/1 -> S-R Flip-Flop1/2
  Right Rescue Function/1(y) -> Relational Operator/2
  Left Rescue Function/1(y) -> Relational Operator3/2
  LlkMt/1 -> Left Catastophe Function/1(u), Left Rescue Function/2(v)
  LrkMt/1 -> Right Catastophe Function/1(u), Right Rescue Function/2(v)
  Fspr/1 -> Left Rescue Function/1(u), Right Rescue Function/1(u)
  S-R Flip-Flop/1 -> CLeft/1
  S-R Flip-Flop/2 -> RLeft/1
  S-R Flip-Flop1/1 -> CRight/1
  S-R Flip-Flop1/2 -> RRight/1

== system Coupled_Model_crosslinked_intext/kMtcontrol/kMtcontrol3/kMt Dynamics /kMtState ==
  LlkMt : Inport
  Fspr : Inport  Port=2
  LrkMt : Inport  Port=3
  Left Catastophe Function : MATLAB Function  TreatAsAtomicUnit=on
  Left Rescue Function : MATLAB Function  TreatAsAtomicUnit=on
  Relational Operator{,1..3} (4 alike) : RelationalOperator  Operator=<=  OutDataTypeStr=boolean
  Right Catastophe Function : MATLAB Function  TreatAsAtomicUnit=on
  Right Rescue Function : MATLAB Function  TreatAsAtomicUnit=on
  S-R Flip-Flop : simulink_extras/Flip Flops/S-R Flip-Flop  SystemSampleTime=-1  initial_condition=0
  S-R Flip-Flop1 : simulink_extras/Flip Flops/S-R Flip-Flop  SystemSampleTime=-1  initial_condition=0
  Uniform Random Number : UniformRandomNumber  Minimum=0  Seed=randi(10000)+1  SampleTime=1
  Uniform Random Number1 : UniformRandomNumber  Minimum=0  Seed=randi(10000)+2  SampleTime=1
  Uniform Random Number2 : UniformRandomNumber  Minimum=0  Seed=randi(10000)+4  SampleTime=1
  Uniform Random Number3 : UniformRandomNumber  Minimum=0  Seed=randi(10000)+3  SampleTime=1
  CLeft : Outport
  RLeft : Outport  Port=2
  CRight : Outport  Port=3
  RRight : Outport  Port=4
  wires:
  Left Catastophe Function/1(y) -> Relational Operator1/2
  Uniform Random Number/1 -> Relational Operator1/1
  Relational Operator1/1 -> S-R Flip-Flop/1
  Right Catastophe Function/1(y) -> Relational Operator2/2
  Uniform Random Number2/1 -> Relational Operator2/1
  Relational Operator2/1 -> S-R Flip-Flop1/1
  Uniform Random Number1/1 -> Relational Operator3/1
  Uniform Random Number3/1 -> Relational Operator/1
  Relational Operator3/1 -> S-R Flip-Flop/2
  Relational Operator/1 -> S-R Flip-Flop1/2
  Right Rescue Function/1(y) -> Relational Operator/2
  Left Rescue Function/1(y) -> Relational Operator3/2
  LlkMt/1 -> Left Catastophe Function/1(u), Left Rescue Function/2(v)
  LrkMt/1 -> Right Catastophe Function/1(u), Right Rescue Function/2(v)
  Fspr/1 -> Left Rescue Function/1(u), Right Rescue Function/1(u)
  S-R Flip-Flop/1 -> CLeft/1
  S-R Flip-Flop/2 -> RLeft/1
  S-R Flip-Flop1/1 -> CRight/1
  S-R Flip-Flop1/2 -> RRight/1

== system Coupled_Model_crosslinked_intext/kMtcontrol/kMtcontrol3/kMt Dynamics  /kMtState ==
  LlkMt : Inport
  Fspr : Inport  Port=2
  LrkMt : Inport  Port=3
  Left Catastophe Function : MATLAB Function  TreatAsAtomicUnit=on
  Left Rescue Function : MATLAB Function  TreatAsAtomicUnit=on
  Relational Operator{,1..3} (4 alike) : RelationalOperator  Operator=<=  OutDataTypeStr=boolean
  Right Catastophe Function : MATLAB Function  TreatAsAtomicUnit=on
  Right Rescue Function : MATLAB Function  TreatAsAtomicUnit=on
  S-R Flip-Flop : simulink_extras/Flip Flops/S-R Flip-Flop  SystemSampleTime=-1  initial_condition=0
  S-R Flip-Flop1 : simulink_extras/Flip Flops/S-R Flip-Flop  SystemSampleTime=-1  initial_condition=0
  Uniform Random Number : UniformRandomNumber  Minimum=0  Seed=randi(10000)+1  SampleTime=1
  Uniform Random Number1 : UniformRandomNumber  Minimum=0  Seed=randi(10000)+2  SampleTime=1
  Uniform Random Number2 : UniformRandomNumber  Minimum=0  Seed=randi(10000)+4  SampleTime=1
  Uniform Random Number3 : UniformRandomNumber  Minimum=0  Seed=randi(10000)+3  SampleTime=1
  CLeft : Outport
  RLeft : Outport  Port=2
  CRight : Outport  Port=3
  RRight : Outport  Port=4
  wires:
  Left Catastophe Function/1(y) -> Relational Operator1/2
  Uniform Random Number/1 -> Relational Operator1/1
  Relational Operator1/1 -> S-R Flip-Flop/1
  Right Catastophe Function/1(y) -> Relational Operator2/2
  Uniform Random Number2/1 -> Relational Operator2/1
  Relational Operator2/1 -> S-R Flip-Flop1/1
  Uniform Random Number1/1 -> Relational Operator3/1
  Uniform Random Number3/1 -> Relational Operator/1
  Relational Operator3/1 -> S-R Flip-Flop/2
  Relational Operator/1 -> S-R Flip-Flop1/2
  Right Rescue Function/1(y) -> Relational Operator/2
  Left Rescue Function/1(y) -> Relational Operator3/2
  LlkMt/1 -> Left Catastophe Function/1(u), Left Rescue Function/2(v)
  LrkMt/1 -> Right Catastophe Function/1(u), Right Rescue Function/2(v)
  Fspr/1 -> Left Rescue Function/1(u), Right Rescue Function/1(u)
  S-R Flip-Flop/1 -> CLeft/1
  S-R Flip-Flop/2 -> RLeft/1
  S-R Flip-Flop1/1 -> CRight/1
  S-R Flip-Flop1/2 -> RRight/1

== matlab function Coupled_Model_crosslinked_intext/kMtcontrol/kMtcontrol1/ Spring Function ==
  data: popped output; Lspr input; F output; thresh input; K1 input
function [popped, F] = fcn(Lspr,thresh,K1)
%#eml

rest=0.2e-6;
popLength=0.45e-6;
springLength=0.8e-6;


K2=K1*springLength/(springLength+popLength);

popped=false;


if Lspr < thresh
    F=K1*(Lspr-rest);
    popped=false;

elseif Lspr >= thresh
    F=K2*(Lspr-rest-popLength);
    popped=true;
    
else
    F=0;
end

end

== matlab function Coupled_Model_crosslinked_intext/ipMtcontrol/Embedded MATLAB Function1 ==
  data: singleipMtIN input; singlekMtIN input; doubleIN input; freeIN input; Lip input; Nmotors output; Llap input; LkMt input
function Nmotors    = tick(singleipMtIN, singlekMtIN, doubleIN, freeIN, Lip, Llap, LkMt)

persistent singleBoundipMt1 singleBoundipMt2 singleBoundipMt3 singleBoundipMt4 singleBoundkMt doubleBound1 doubleBound2 doubleBound3 doubleBound4 unBound
if isempty(singleBoundipMt1) && isempty(singleBoundipMt2) && isempty(singleBoundipMt3) && isempty(singleBoundipMt4) && isempty(singleBoundkMt) && isempty(doubleBound1) && isempty(doubleBound2)&& isempty(doubleBound3)&& isempty(doubleBound3)&& isempty(doubleBound4) && isempty(unBound)
    singleBoundipMt1 = singleipMtIN; 
    singleBoundipMt2 = singleipMtIN;
    singleBoundipMt3 = singleipMtIN;
    singleBoundipMt4 = singleipMtIN;
    singleBoundkMt = singlekMtIN;
    doubleBound1 = doubleIN;
    doubleBound2 = doubleIN;
    doubleBound3 = doubleIN;
    doubleBound4 = doubleIN;
    unBound = freeIN;
    Nmotors = doubleBound1+doubleBound2+doubleBound3+doubleBound4;
%     singleipMt1 = singleBoundipMt1;
%     singleipMt2 = singleBoundipMt2;
%     singleipMt3 = singleBoundipMt3;
%     singleipMt4 = singleBoundipMt4;
%     singlekMt = singleBoundkMt;
%     free = unBound;
else
    
% double bound motors detaching    
    off = @doubleToSingle;
    doubleOff1 = off(doubleBound1);
    doubleOff2 = off(doubleBound2);
    doubleOff3 = off(doubleBound3);
    doubleOff4 = off(doubleBound4);
    
% double bound motors attaching
    on = @singleToDouble;
    doubleOn1 = on(singleBoundipMt1, Llap, Lip);
    doubleOn2 = on(singleBoundipMt2, Llap, Lip);
    doubleOn3 = on(singleBoundipMt3, Llap, Lip);
    doubleOn4 = on(singleBoundipMt4, Llap, Lip);
    
% single bound motors attaching  
    onipMt = @freeToSingleipMt;
    singleOnipMt1 = onipMt(unBound, Lip, Llap, LkMt);
    singleOnipMt2 = onipMt(unBound, Lip, Llap, LkMt);
    singleOnipMt3 = onipMt(unBound, Lip, Llap, LkMt);
    singleOnipMt4 = onipMt(unBound, Lip, Llap, LkMt);
    
    onkMt = @freeToSinglekMt;
    singleOnkMt = onkMt(unBound, Lip, Llap, LkMt);
    
% single bound motors detaching
    off = @singleToFree;
    singleOffipMt1 = off(singleBoundipMt1);
    singleOffipMt2 = off(singleBoundipMt2);
    singleOffipMt3 = off(singleBoundipMt3);
    singleOffipMt4 = off(singleBoundipMt4);
    
    singleOffkMt = off(singleBoundkMt);
    
% calculate net on and off 
    % currently assuming that double attached motors go to singly attached motors
    doubleBound1 = doubleBound1 + doubleOn1 - doubleOff1;
    doubleBound2 = doubleBound2 + doubleOn2 - doubleOff2;
    doubleBound3 = doubleBound3 + doubleOn3 - doubleOff3;
    doubleBound4 = doubleBound4 + doubleOn4 - doubleOff4;
    singleBoundipMt1 = singleBoundipMt1 + singleOnipMt1 - singleOffipMt1 + doubleOff1 - doubleOn1;
    singleBoundipMt2 = singleBoundipMt2 + singleOnipMt2 - singleOffipMt2 + doubleOff2 - doubleOn2;
    singleBoundipMt3 = singleBoundipMt3 + singleOnipMt3 - singleOffipMt3 + doubleOff3 - doubleOn3;
    singleBoundipMt4 = singleBoundipMt4 + singleOnipMt4 - singleOffipMt4 + doubleOff4 - doubleOn4;
    singleBoundkMt = singleBoundkMt +singleOnkMt - singleOffkMt;
    unBound = unBound + singleOffipMt1 + singleOffipMt2 + singleOffipMt3 + singleOffipMt4 + singleOffkMt- singleOnipMt1 - singleOnipMt2 - singleOnipMt3 - singleOnipMt4 - singleOnkMt;
% assignment to output variables
    Nmotors = doubleBound1+doubleBound2+doubleBound3+doubleBound4;
%     singlekMt = singleBoundkMt;
%     singleipMt1 = singleBoundipMt1;
%     singleipMt2 = singleBoundipMt2;
%     singleipMt3 = singleBoundipMt3;
%     singleipMt4 = singleBoundipMt4;
%     free = unBound;
end

== matlab function Coupled_Model_crosslinked_intext/kMtcontrol/kMtcontrol1/ Spring Function  ==
  data: popped output; Lspr input; F output; thresh input; K1 input
function [popped, F] = fcn(Lspr,thresh,K1)
%#eml

rest=0.2e-6;
popLength=0.45e-6;
springLength=0.8e-6;


K2=K1*springLength/(springLength+popLength);

popped=false;


if Lspr < thresh
    F=K1*(Lspr-rest);
    popped=false;

elseif Lspr >= thresh
    F=K2*(Lspr-rest-popLength);
    popped=true;
    
else
    F=0;
end

end

== matlab function Coupled_Model_crosslinked_intext/kMtcontrol/kMtcontrol1/Spring Function ==
  data: popped output; Lspr input; F output; thresh input; K1 input
function [popped, F] = fcn(Lspr,thresh,K1)
%#eml

rest=0.2e-6;
popLength=0.45e-6;
springLength=0.8e-6;


K2=K1*springLength/(springLength+popLength);

popped=false;


if Lspr < thresh
    F=K1*(Lspr-rest);
    popped=false;

elseif Lspr >= thresh
    F=K2*(Lspr-rest-popLength);
    popped=true;
    
else
    F=0;
end

end

== matlab function Coupled_Model_crosslinked_intext/kMtcontrol/kMtcontrol1/Spring Function  ==
  data: popped output; Lspr input; F output; thresh input; K1 input
function [popped, F] = fcn(Lspr,thresh,K1)
%#eml

rest=0.2e-6;
popLength=0.45e-6;
springLength=0.8e-6;


K2=K1*springLength/(springLength+popLength);

popped=false;


if Lspr < thresh
    F=K1*(Lspr-rest);
    popped=false;

elseif Lspr >= thresh
    F=K2*(Lspr-rest-popLength);
    popped=true;
    
else
    F=0;
end

end

== matlab function Coupled_Model_crosslinked_intext/kMtcontrol/kMtcontrol1/kMt  Dynamics/kMtState/Left Catastophe Function ==
  data: u input; y output
function y = fcn(u)
%#eml
if u < 8e-7
y = -.65*((u*10^6)-0.75).^2+(23/60);
else 
    y=0.389;
end
y=abs(y);

== matlab function Coupled_Model_crosslinked_intext/kMtcontrol/kMtcontrol1/kMt  Dynamics/kMtState/Left Rescue Function ==
  data: u input; y output; v input
function y = fcn(u,v)
%#eml
if v<=0.05e-6
    y=1;
else
    y=-9.5e9*(u)+0.21;
end
y=abs(y);

== matlab function Coupled_Model_crosslinked_intext/kMtcontrol/kMtcontrol1/kMt  Dynamics/kMtState/Right Catastophe Function ==
  data: u input; y output
function y = fcn(u)
%#eml
if u < 8e-7
y = -.65*((u*10^6)-0.75).^2+(23/60);
else 
    y=.389;
end
y=abs(y);

== matlab function Coupled_Model_crosslinked_intext/kMtcontrol/kMtcontrol1/kMt  Dynamics/kMtState/Right Rescue Function ==
  data: u input; y output; v input
function y = fcn(u,v)
%#eml
if v<=0.05e-6
    y=1;
else
    y=-9.5e9*(u)+0.21;
end
y=abs(y);

== matlab function Coupled_Model_crosslinked_intext/kMtcontrol/kMtcontrol1/kMt Dynamics/kMtState/Left Catastophe Function ==
  data: u input; y output
function y = fcn(u)
%#eml
if u < 8e-7
y = -.65*((u*10^6)-0.75).^2+(23/60);
else 
    y=0.389;
end
y=abs(y);

== matlab function Coupled_Model_crosslinked_intext/kMtcontrol/kMtcontrol1/kMt Dynamics/kMtState/Left Rescue Function ==
  data: u input; y output; v input
function y = fcn(u,v)
%#eml
if v<=0.05e-6
    y=1;
else
    y=-9.5e9*(u)+0.21;
end
y=abs(y);

== matlab function Coupled_Model_crosslinked_intext/kMtcontrol/kMtcontrol1/kMt Dynamics/kMtState/Right Catastophe Function ==
  data: u input; y output
function y = fcn(u)
%#eml
if u < 8e-7
y = -.65*((u*10^6)-0.75).^2+(23/60);
else 
    y=.389;
end
y=abs(y);

== matlab function Coupled_Model_crosslinked_intext/kMtcontrol/kMtcontrol1/kMt Dynamics/kMtState/Right Rescue Function ==
  data: u input; y output; v input
function y = fcn(u,v)
%#eml
if v<=0.05e-6
    y=1;
else
    y=-9.5e9*(u)+0.21;
end
y=abs(y);

== matlab function Coupled_Model_crosslinked_intext/kMtcontrol/kMtcontrol1/kMt Dynamics /kMtState/Left Catastophe Function ==
  data: u input; y output
function y = fcn(u)
%#eml
if u < 8e-7
y = -.65*((u*10^6)-0.75).^2+(23/60);
else 
    y=0.389;
end
y=abs(y);

== matlab function Coupled_Model_crosslinked_intext/kMtcontrol/kMtcontrol1/kMt Dynamics /kMtState/Left Rescue Function ==
  data: u input; y output; v input
function y = fcn(u,v)
%#eml
if v<=0.05e-6
    y=1;
else
    y=-9.5e9*(u)+0.21;
end
y=abs(y);

== matlab function Coupled_Model_crosslinked_intext/kMtcontrol/kMtcontrol1/kMt Dynamics /kMtState/Right Catastophe Function ==
  data: u input; y output
function y = fcn(u)
%#eml
if u < 8e-7
y = -.65*((u*10^6)-0.75).^2+(23/60);
else 
    y=.389;
end
y=abs(y);

== matlab function Coupled_Model_crosslinked_intext/kMtcontrol/kMtcontrol1/kMt Dynamics /kMtState/Right Rescue Function ==
  data: u input; y output; v input
function y = fcn(u,v)
%#eml
if v<=0.05e-6
    y=1;
else
    y=-9.5e9*(u)+0.21;
end
y=abs(y);

== matlab function Coupled_Model_crosslinked_intext/kMtcontrol/kMtcontrol1/kMt Dynamics  /kMtState/Left Catastophe Function ==
  data: u input; y output
function y = fcn(u)
%#eml
if u < 8e-7
y = -.65*((u*10^6)-0.75).^2+(23/60);
else 
    y=0.389;
end
y=abs(y);

== matlab function Coupled_Model_crosslinked_intext/kMtcontrol/kMtcontrol1/kMt Dynamics  /kMtState/Left Rescue Function ==
  data: u input; y output; v input
function y = fcn(u,v)
%#eml
if v<=0.05e-6
    y=1;
else
    y=-9.5e9*(u)+0.21;
end
y=abs(y);

== matlab function Coupled_Model_crosslinked_intext/kMtcontrol/kMtcontrol1/kMt Dynamics  /kMtState/Right Catastophe Function ==
  data: u input; y output
function y = fcn(u)
%#eml
if u < 8e-7
y = -.65*((u*10^6)-0.75).^2+(23/60);
else 
    y=.389;
end
y=abs(y);

== matlab function Coupled_Model_crosslinked_intext/kMtcontrol/kMtcontrol1/kMt Dynamics  /kMtState/Right Rescue Function ==
  data: u input; y output; v input
function y = fcn(u,v)
%#eml
if v<=0.05e-6
    y=1;
else
    y=-9.5e9*(u)+0.21;
end
y=abs(y);

== matlab function Coupled_Model_crosslinked_intext/Polcontrol/Embedded MATLAB Function1 ==
  data: Fnet input; y output; Nmotors input
function y = fcn(Fnet,Nmotors)
%#eml
if Nmotors == 0
    y = 0;
else
    y = Fnet/Nmotors;
end

== matlab function Coupled_Model_crosslinked_intext/Polcontrol/Embedded MATLAB Function ==
  data: Fnet input; Vip output
function Vip=fcn(Fnet)
%#eml

% if Fnet < 6e-12
    Vip=(50e-9/6e-12)*Fnet;
% else
%     Vip=50e-9;
% end

== matlab function Coupled_Model_crosslinked_intext/kMtcontrol/kMtcontrol2/ Spring Function ==
  data: popped output; Lspr input; F output; thresh input; K1 input
function [popped, F] = fcn(Lspr,thresh,K1)
%#eml

rest=0.2e-6;
popLength=0.45e-6;
springLength=0.8e-6;


K2=K1*springLength/(springLength+popLength);

popped=false;


if Lspr < thresh
    F=K1*(Lspr-rest);
    popped=false;

elseif Lspr >= thresh
    F=K2*(Lspr-rest-popLength);
    popped=true;
    
else
    F=0;
end

end

== matlab function Coupled_Model_crosslinked_intext/kMtcontrol/kMtcontrol2/ Spring Function  ==
  data: popped output; Lspr input; F output; thresh input; K1 input
function [popped, F] = fcn(Lspr,thresh,K1)
%#eml

rest=0.2e-6;
popLength=0.45e-6;
springLength=0.8e-6;


K2=K1*springLength/(springLength+popLength);

popped=false;


if Lspr < thresh
    F=K1*(Lspr-rest);
    popped=false;

elseif Lspr >= thresh
    F=K2*(Lspr-rest-popLength);
    popped=true;
    
else
    F=0;
end

end
